simulink model "modelo_simplificado"  (R2023b)
settings: Solver=VariableStepAuto  StartTime=0.0  StopTime=10.0  MaxStep=0.001  RelTol=1e-3
values from neighbouring files (symbols this model uses):
  frac_polar = [0 0.01 0.02 0.03 0.04 0.05 0.06 0.07 0.08 0.09 0.1 0.11 ... (201 elements, 201x1)]    [CargaDatosLSM.mat]
  fuerza = [171.672724896 186.73762089 200.980211078 214.312162114 226.676669826 238.025601636 248.273052104 257.388258855 265.32487317 272.007156436 277.296044751 280.812078814 ... (24321 elements, 121x201)]    [CargaDatosLSM.mat]    (also in dinamica_LSM.mat = [0 0 520.6454518 510.814195972 501.0938194 493.204723564 485)
undefined symbols (not defined in the file or in its folder): angulo, DiscIntNeverNeededParam
settings Model: Creator=USUARIO  LastModifiedBy=USUARIO

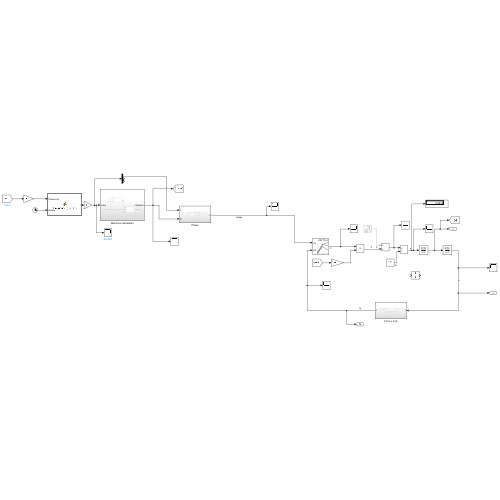
[thumbnail: Simulink's stored preview of the top-level diagram]
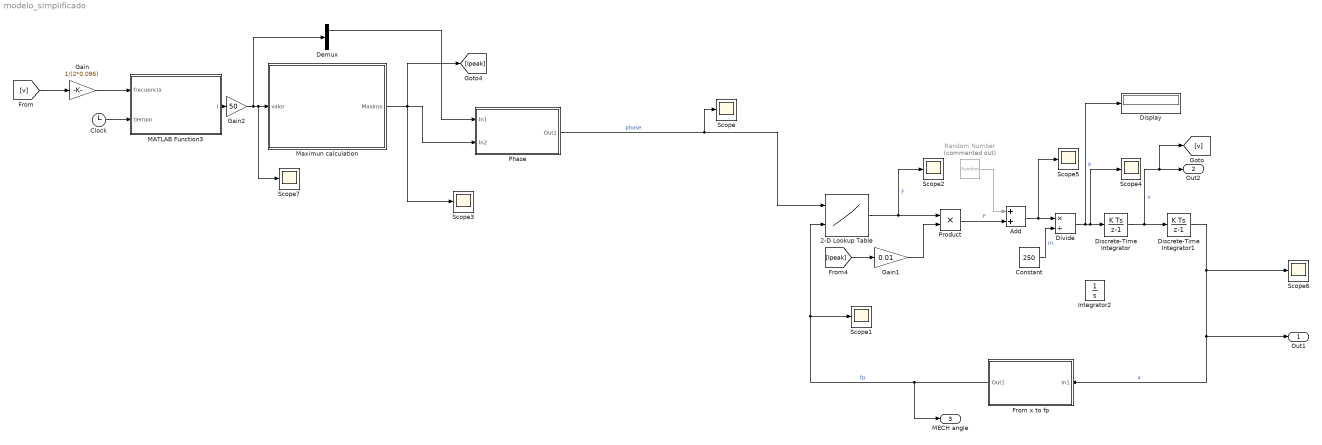
== system modelo_simplificado ==
  2-D Lookup Table : Lookup_n-D  BreakpointsForDimension1=angulo  BreakpointsForDimension2=frac_polar  Table=fuerza  InternalRulePriority=Speed  RndMeth=Simplest
      settings: InputPortMap=u0,u1
  Add : Sum
  Clock : Clock
  Constant : Constant  Value=250
  Demux : Demux  Outputs=3
  Discrete-Time Integrator : DiscreteIntegrator  InitialCondition=1  SampleTime=-1  ICPrevOutput=DiscIntNeverNeededParam  ICPrevScaledInput=DiscIntNeverNeededParam
  Discrete-Time Integrator1 : DiscreteIntegrator  SampleTime=-1  ICPrevOutput=DiscIntNeverNeededParam  ICPrevScaledInput=DiscIntNeverNeededParam
  Display : Display
  Divide : Product  Inputs=*/
  From x to fp : Subsystem
  Gain : Gain  Gain=1/(2*0.096)
  Gain1 : Gain  Gain=0.01
  Gain2 : Gain  Gain=50
  Integrator2 : Integrator
  MATLAB Function3 : MATLAB Function  TreatAsAtomicUnit=on
  Maximun calculation : Subsystem
  Phase : Subsystem
  Product : Product
  Random Number : RandomNumber  Commented=on  Mean=-10  SampleTime=0.1
  Scope{,1..7} (8 alike) : Scope
  Out1 : Outport
  Out2 : Outport  Port=2
  MECH angle : Outport  Port=3
  wires:
  Discrete-Time Integrator/1 -> Discrete-Time Integrator1/1, [v], Out2/1  "v"
  Discrete-Time Integrator1/1 -> Out1/1, From x to fp/1(In1), Scope6/1  "x"
  Constant/1 -> Divide/2  "m"
  Gain2/1 -> Demux/1, Scope7/1, Maximun calculation/1(valor)
  [Ipeak] -> Gain1/1
  Demux/1 -> Phase/1(In1)
  Gain1/1 -> Product/2
  2-D Lookup Table/1 -> Scope2/1, Product/1  "F"
  From x to fp/1(Out1) -> MECH angle/1, Scope1/1, 2-D Lookup Table/2  "fp"
  Phase/1(Out1) -> Scope/1, 2-D Lookup Table/1  "phase"
  Maximun calculation/1(Maximo) -> [Ipeak], Scope3/1, Phase/2(In2)
  Add/1 -> Scope5/1, Divide/1
  Divide/1 -> Display/1, Discrete-Time Integrator/1, Scope4/1  "a"
  Random Number/1 -> Add/1
  Product/1 -> Add/2  "F"
  Clock/1 -> MATLAB Function3/2(tiempo)
  [v] -> Gain/1
  Gain/1 -> MATLAB Function3/1(frecuencia)
  MATLAB Function3/1(i) -> Gain2/1

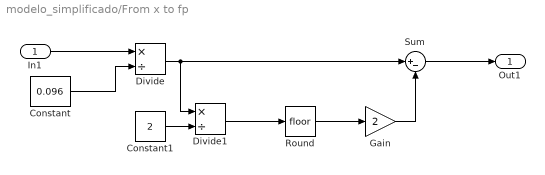
== system modelo_simplificado/From x to fp ==
  In1 : Inport
  Constant : Constant  Value=0.096
  Constant1 : Constant  Value=2
  Divide : Product  Inputs=*/
  Divide1 : Product  Inputs=*/
  Gain : Gain  Gain=2
  Round : Rounding
  Sum : Sum  Inputs=|+-
  Out1 : Outport
  wires:
  In1/1 -> Divide/1
  Constant/1 -> Divide/2
  Divide/1 -> Divide1/1, Sum/1
  Divide1/1 -> Round/1
  Round/1 -> Gain/1
  Constant1/1 -> Divide1/2
  Gain/1 -> Sum/2
  Sum/1 -> Out1/1

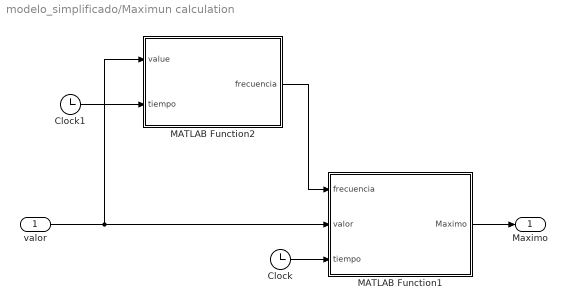
== system modelo_simplificado/Maximun calculation ==
  valor : Inport
  Clock : Clock
  Clock1 : Clock
  MATLAB Function1 : MATLAB Function  TreatAsAtomicUnit=on
  MATLAB Function2 : MATLAB Function  TreatAsAtomicUnit=on
  Maximo : Outport
  wires:
  valor/1 -> MATLAB Function2/1(value), MATLAB Function1/2(valor)
  Clock/1 -> MATLAB Function1/3(tiempo)
  MATLAB Function2/1(frecuencia) -> MATLAB Function1/1(frecuencia)
  Clock1/1 -> MATLAB Function2/2(tiempo)
  MATLAB Function1/1(Maximo) -> Maximo/1

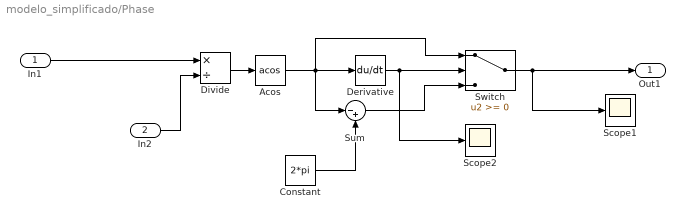
== system modelo_simplificado/Phase ==
  In1 : Inport
  In2 : Inport  Port=2
  Acos : Trigonometry  Operator=acos
  Constant : Constant  Value=2*pi
  Derivative : Derivative
  Divide : Product  Inputs=*/
  Scope1 : Scope
  Scope2 : Scope
  Sum : Sum  Inputs=|-+
  Switch : Switch  SaturateOnIntegerOverflow=off  InputSameDT=off
  Out1 : Outport
  wires:
  In1/1 -> Divide/1
  Derivative/1 -> Scope2/1, Switch/2
  Acos/1 -> Switch/1, Sum/1, Derivative/1
  Sum/1 -> Switch/3
  Switch/1 -> Out1/1, Scope1/1
  Constant/1 -> Sum/2
  In2/1 -> Divide/2
  Divide/1 -> Acos/1

== matlab function modelo_simplificado/Maximun calculation/MATLAB Function1 ==
  settings: updateMethod=DISCRETE
  data: frecuencia input; Maximo output; valor input; tiempo input
function Maximo = fcn(frecuencia,valor,tiempo)

   persistent antiguo_maximo
    if isempty(antiguo_maximo)
       antiguo_maximo=0;
    end
    persistent t_maximo
    if isempty(t_maximo)
       t_maximo=0;
    end

maximo = [0 0 0];

periodo=1/abs(frecuencia)/3;

for i=1:3
    if abs(valor(i))>=antiguo_maximo
        maximo(i)=abs(valor(i));
        antiguo_maximo=abs(valor(i));
        t_maximo=tiempo;
    else
        maximo(i)=antiguo_maximo;
        if tiempo>t_maximo+periodo
            maximo(i)=abs(valor(i));
            antiguo_maximo=abs(valor(i));
            t_maximo=tiempo;
        end
    end
end

Maximo = max(maximo);

== matlab function modelo_simplificado/Maximun calculation/MATLAB Function2 ==
  settings: updateMethod=DISCRETE
  data: frecuencia output; value input; tiempo input
function frecuencia = frecuency_calculator(value,tiempo)

   persistent signo
    if isempty(signo)
       signo=[0 0 0]; % 1 positive, 2 negative
    end
    persistent t_inicio
    if isempty(t_inicio)
       t_inicio=[0 0 0];
    end

    persistent frecuencia_acc
    if isempty(frecuencia_acc)
       frecuencia_acc=1;
    end

    frecuencia=frecuencia_acc;

    for i=1:3
    
        if signo(i) == 0
            if value(i) >= 0 
                signo(i) = 1;
            else
                signo(i) = 2;
            end
            t_inicio(i)=tiempo;
        end
        
        if signo(i)==1
            if value(i) <= 0
                frecuencia = 1/(2*(tiempo-t_inicio(i)));
                frecuencia_acc=frecuencia;
                signo(i) = 0;
            end
        end
        
        if signo(i)==2
            if value(i) >= 0
                frecuencia = 1/(2*(tiempo-t_inicio(i)));
                frecuencia_acc=frecuencia;
                signo(i) = 0;
            end
        end

    end

== matlab function modelo_simplificado/MATLAB Function3 ==
  settings: updateMethod=DISCRETE
  data: i output; frecuencia input; tiempo input
function i = three_phase_generator(frecuencia, tiempo)
persistent fase
    if isempty(fase)
        fase=0;
    end
persistent t_1
    if isempty(t_1)
        t_1=0;
    end
periodo = 1/frecuencia;
dt = tiempo-t_1;
dfase = dt/periodo*2*pi;
fase = fase + dfase;
if fase>=2*pi
    fase=0;
end
u = sin(fase);
v = sin(fase + 2*pi/3);
w = sin(fase + 4*pi/3);
i = [u, v, w];
t_1=tiempo;
